simulink model "zbiorniki_objekt"  (R2021b)
settings: Solver=FixedStepDiscrete  StartTime=0.0  StopTime=10.0  FixedStep=0.1  RelTol=1e-3
values from neighbouring files (symbols this model uses):
  a1 = 10    [Parametry_objektu.m]
  a2 = 10    [Parametry_objektu.m]
  c1 = 35    [Parametry_objektu.m]
  c2 = 32    [Parametry_objektu.m]
  p = 0    [Parametry_objektu.m]
  q = 100    [Parametry_objektu.m]
  v1 = 1    [Parametry_objektu.m]
  v2 = 1    [Parametry_objektu.m]
undefined symbols (not defined in the file or in its folder): DiscIntNeverNeededParam
settings Model: Creator=lab  LastModifiedBy=lab
settings ConfigComp: PLC_TargetIDE=plcopen  PLC_MultiTBSigbuilderTimeRange=off  PLC_InlineEnumCastFunction=off

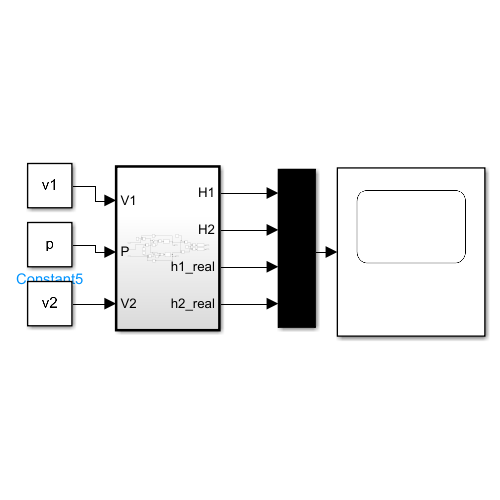
[thumbnail: Simulink's stored preview of the top-level diagram]
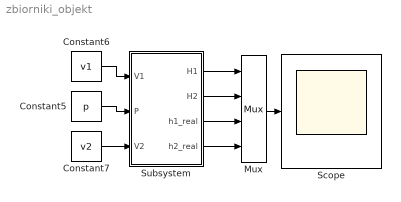
== system zbiorniki_objekt ==
  Constant5 : Constant  Value=p  OutDataTypeStr=boolean
  Constant6 : Constant  Value=v1  OutDataTypeStr=boolean
  Constant7 : Constant  Value=v2  OutDataTypeStr=boolean
  Mux : Mux
  Scope : Scope
  Subsystem : Subsystem  TreatAsAtomicUnit=on
  wires:
  Mux/1 -> Scope/1
  Constant6/1 -> Subsystem/1(V1)
  Constant5/1 -> Subsystem/2(P)
  Constant7/1 -> Subsystem/3(V2)
  Subsystem/1(H1) -> Mux/1
  Subsystem/2(H2) -> Mux/2
  Subsystem/3(h1_real) -> Mux/3
  Subsystem/4(h2_real) -> Mux/4

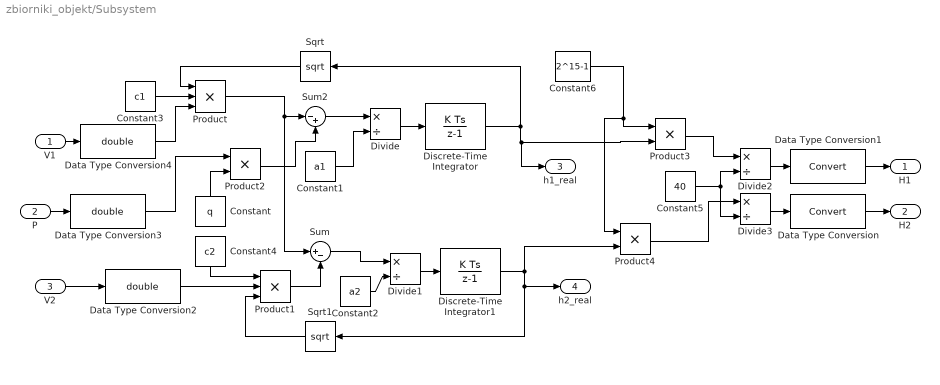
== system zbiorniki_objekt/Subsystem ==
  V1 : Inport  OutDataTypeStr=boolean
  P : Inport  Port=2  OutDataTypeStr=boolean
  V2 : Inport  Port=3  OutDataTypeStr=boolean
  Constant : Constant  Value=q
  Constant1 : Constant  Value=a1
  Constant2 : Constant  Value=a2
  Constant3 : Constant  Value=c1
  Constant4 : Constant  Value=c2
  Constant5 : Constant  Value=40
  Constant6 : Constant  Value=2^15-1  OutDataTypeStr=double
  Data Type Conversion : DataTypeConversion
  Data Type Conversion1 : DataTypeConversion
  Data Type Conversion2 : DataTypeConversion  OutDataTypeStr=double
  Data Type Conversion3 : DataTypeConversion  OutDataTypeStr=double
  Data Type Conversion4 : DataTypeConversion  OutDataTypeStr=double
  Discrete-Time Integrator : DiscreteIntegrator  SampleTime=-1  OutDataTypeStr=double  LimitOutput=on  UpperSaturationLimit=40  LowerSaturationLimit=0  ICPrevOutput=DiscIntNeverNeededParam  ICPrevScaledInput=DiscIntNeverNeededParam
  Discrete-Time Integrator1 : DiscreteIntegrator  SampleTime=-1  LimitOutput=on  UpperSaturationLimit=40  LowerSaturationLimit=0  ICPrevOutput=DiscIntNeverNeededParam  ICPrevScaledInput=DiscIntNeverNeededParam
  Divide{,1..3} (4 alike) : Product  Inputs=*/
  Product : Product  Inputs=3
  Product1 : Product  Inputs=3
  Product2 : Product
  Product3 : Product
  Product4 : Product
  Sqrt : Sqrt  SaturateOnIntegerOverflow=on
  Sqrt1 : Sqrt  SaturateOnIntegerOverflow=on
  Sum : Sum  Inputs=|+-
  Sum2 : Sum  Inputs=|-+
  H1 : Outport  OutDataTypeStr=uint16
  H2 : Outport  Port=2  OutDataTypeStr=uint16
  h1_real : Outport  Port=3
  h2_real : Outport  Port=4
  wires:
  Product/1 -> Sum/1, Sum2/1
  Sum/1 -> Divide1/1
  Sum2/1 -> Divide/1
  Constant3/1 -> Product/2
  Product1/1 -> Sum/2
  Constant/1 -> Product2/2
  Sqrt/1 -> Product/1
  Constant4/1 -> Product1/1
  Sqrt1/1 -> Product1/3
  Constant1/1 -> Divide/2
  Constant2/1 -> Divide1/2
  Product2/1 -> Sum2/2
  Divide/1 -> Discrete-Time Integrator/1
  Discrete-Time Integrator/1 -> Product3/2, h1_real/1, Sqrt/1
  Divide1/1 -> Discrete-Time Integrator1/1
  Discrete-Time Integrator1/1 -> h2_real/1, Sqrt1/1, Product4/2
  Divide3/1 -> Data Type Conversion/1
  Constant5/1 -> Divide3/2, Divide2/2
  Constant6/1 -> Product4/1, Product3/1
  Product3/1 -> Divide2/1
  Data Type Conversion/1 -> H2/1
  Divide2/1 -> Data Type Conversion1/1
  Data Type Conversion1/1 -> H1/1
  Product4/1 -> Divide3/1
  Data Type Conversion2/1 -> Product1/2
  V2/1 -> Data Type Conversion2/1
  V1/1 -> Data Type Conversion4/1
  Data Type Conversion4/1 -> Product/3
  P/1 -> Data Type Conversion3/1
  Data Type Conversion3/1 -> Product2/1
